simulink library "lib_Convection_SimpConvHeatX"  (R2015a)
settings: Solver=ode45  StartTime=0.0  StopTime=10.0  RelTol=1e-3
settings Model: Creator=jlkratz  LastModifiedBy=jlkratz

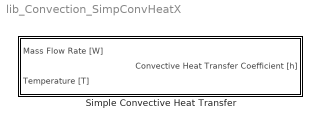
== system lib_Convection_SimpConvHeatX ==
  Simple Convective Heat Transfer : Subsystem  mask(Simple Convective Heat Transfer Block (T-SAT)){hcoeff_M=0.03, Wdes_M=1, TempDep_M=on, Tdes_M=1, BN_M=gcb}
      mask prompts: hcoeff_M "hcoeff_M - Convective heat transfer coefficient when W = Wdes and T = Tdes"; Wdes_M "Wdes_M - Design mass flow rate (known data point)"; TempDep_M "TempDep_M - Temperature effects (checked - include temperature, unchecked - neglect temperture)"; Tdes_M "Tdes_M - Design temperature (known data point)"; BN_M "BN_M - Block name"
      mask help:
      | This block models takes a simplistic apporach at modeling the convective heat transfer coefficient (h) of an internal flow. The equation for calculating the convective heat transfer coefficient is based on empirical models and attempts to correlate the heat transfer coefficient with mass flow rate (W) and the fluid temperature (T).
      |
      | h = hcoeff * (T/Tdes)^0.23 * (W/Wdes)^0.8
      |
      | In the equation above, Tdes and Wdes are the temperautre and mass flow rate of the fluid when h = hcoeff. This block can accept various units but the units must be consistent (Ex. if Wdes is in slug/sec then W must be in slug/sec, if Tdes is in degR then T must be in degR, and if hcoeff is in (Btu/(sec-ft^2-degR)) then the output h will be in (Btu/(sec-ft^2-degR))).
      mask init:
      | if TempDep_M == 1
      |     if strcmp(get_param([BN_M '/Temperature [T]'],'BlockType'),'Constant')
      |         MSK_ReplaceBlock_TSAT([BN_M '/Temperature [T]'],'built-in/Inport');
      |     end
      |     set_param([BN_M '/Temperature [T]'],'Port','2');
      | elseif TempDep_M == 0
      |     if strcmp(get_param([BN_M '/Temperature [T]'],'BlockType'),'Inport')
      |         MSK_ReplaceBlock_TSAT([BN_M '/Temperature [T]'],'built-in/Constant');
      |         set_param([BN_M '/Temperature [T]'],'Value','Tdes_M');
      |     end
      | end
      mask Help: web(which('Convection_TSAT_SimpConvHeatX.html'),'-helpbrowser')
      mask Callback TempDep_M: MSK_SEC_Enables_TMATS('TempDep_M',4,'en')

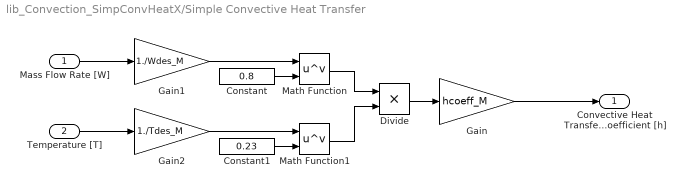
== system lib_Convection_SimpConvHeatX/Simple Convective Heat Transfer ==
  "Mass Flow Rate [W] " : Inport
  Temperature [T] : Inport  Port=2
  Constant : Constant  Value=0.8
  Constant1 : Constant  Value=0.23
  Divide : Product  Inputs=**
  Gain : Gain  Gain=hcoeff_M
  Gain1 : Gain  Gain=1./Wdes_M
  Gain2 : Gain  Gain=1./Tdes_M
  Math Function : Math  Operator=pow  SaturateOnIntegerOverflow=on
  Math Function1 : Math  Operator=pow  SaturateOnIntegerOverflow=on
  Convective Heat Transfer Coefficient [h] : Outport
  wires:
  "Mass Flow Rate [W] "/1 -> Gain1/1
  Constant1/1 -> Math Function1/2
  Math Function1/1 -> Divide/2
  Divide/1 -> Gain/1
  Temperature [T]/1 -> Gain2/1
  Gain/1 -> Convective Heat Transfer Coefficient [h]/1
  Math Function/1 -> Divide/1
  Gain2/1 -> Math Function1/1
  Constant/1 -> Math Function/2
  Gain1/1 -> Math Function/1
